simulink model "vsc_3w_l_filter"  (Simulink 8.9)
settings: Solver=ode23t  StartTime=0.0  StopTime=1  FixedStep=100.0e-6  RelTol=1e-6
values from neighbouring files (symbols this model uses):
  C_dc = 1e6    (= 1000000)    [ini_vsc_3w_l.m]
  F_b = 50.0    (= 50)    [ini_vsc_3w_l.m]
  K_i = R_s/tau_ref    (= 40)    [ini_vsc_3w_l.m]
  K_p = L_s/tau_ref    (= 0.5)    [ini_vsc_3w_l.m]
  L_s = 2.5e-3    (= 0.0025)    [ini_vsc_3w_l.m]
  R_s = 0.2    [ini_vsc_3w_l.m]
  V_dc = 730.0    (= 730)    [ini_vsc_3w_l.m]
  vsc_ctrl_ini = [0,0]    [ini_vsc_3w_l.m]
  vsc_ini = [0,0,V_dc]    [ini_vsc_3w_l.m]
libraries: powerlib x8, powerlib_meascontrol x3
settings Model: Creator=jmmauricio  LastModifiedBy=jmmauricio
settings SolverCC: AlgebraicLoopSolver=LineSearch
settings DataIOCC: LimitDataPoints=off  SaveFormat=Dataset  SignalLoggingSaveFormat=Dataset
settings DebuggingCC: UnderspecifiedInitializationDetection=Simplified  MergeDetectMultiDrivingBlocksExec=error  FcnCallInpInsideContextMsg=error  StateNameClashWarn=none  SFUnexpectedBacktrackingDiag=error  SFNoUnconditionalDefaultTransitionDiag=error
settings HardwareCC: ProdBitPerPointer=64  ProdBitPerSizeT=64  ProdBitPerPtrDiffT=64  ProdLargestAtomicFloat=Float  ProdIntDivRoundTo=Zero  ProdEndianess=LittleEndian  ProdWordSize=64  ProdHWDeviceType=Intel->x86-64 (Windows64)
settings ModelReferenceCC: PropagateSignalLabelsOutOfModel=on
settings GRTTargetCC: TargetLangStandard=C99 (ISO)  GeneratePreprocessorConditionals=Use local settings  CombineOutputUpdateFcns=on  GRTInterface=off
settings ConfigComp: CovMetricSettings=dwe  CovHtmlReporting=off  CovSaveCumulativeToWorkspaceVar=off  CovSaveSingleToWorkspaceVar=off  CovExternalEMLEnable=on

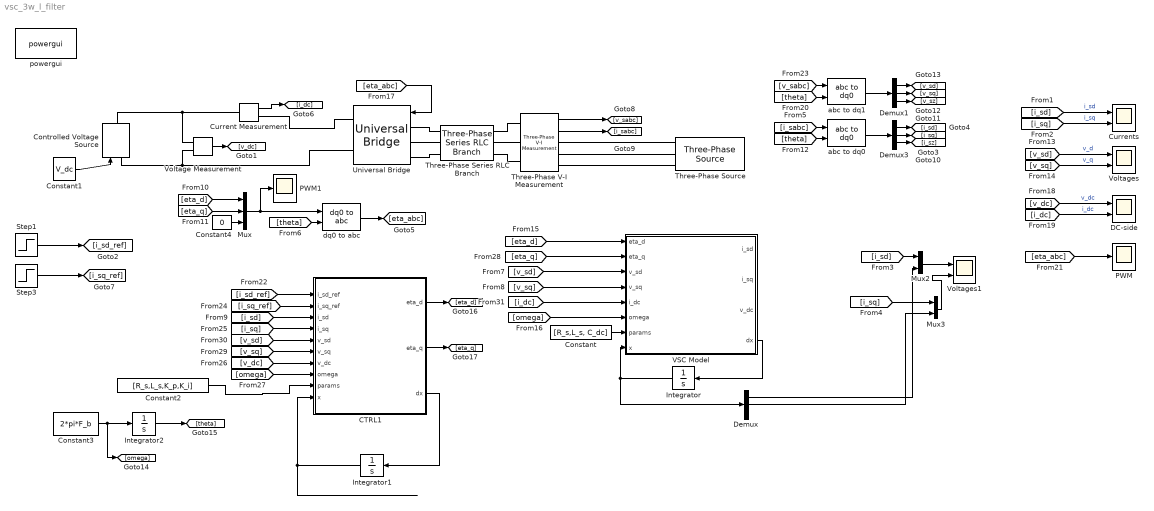
== system vsc_3w_l_filter ==
  CTRL1 : MATLAB Function  TreatAsAtomicUnit=on
  Constant : Constant  Value=[R_s,L_s, C_dc]
  Constant1 : Constant  Value=V_dc
  Constant2 : Constant  Value=[R_s,L_s,K_p,K_i]
  Constant3 : Constant  Value=2*pi*F_b
  Constant4 : Constant  Value=0
  Controlled Voltage Source : powerlib/Electrical Sources/Controlled Voltage Source  Initialize=on  Source_Type=AC  Amplitude=0  Phase=0  Frequency=0  Measurements=None
  Current Measurement : powerlib/Measurements/Current Measurement  PhasorSimulation=off  OutputType=Complex  PSBequivalent=0
  Currents : Scope  NumInputPorts=2
  DC-side : Scope  NumInputPorts=2
  Demux : Demux  Outputs=3
  Demux1 : Demux  Outputs=3
  Demux3 : Demux  Outputs=3
  Integrator : Integrator  InitialCondition=vsc_ini
  Integrator1 : Integrator  InitialCondition=vsc_ctrl_ini
  Integrator2 : Integrator
  Mux : Mux  Inputs=3
  Mux2 : Mux  Inputs=2
  Mux3 : Mux  Inputs=2
  PWM : Scope
  PWM1 : Scope
  Step1 : Step  Time=0.1  After=100  SampleTime=0
  Step3 : Step  Time=0.15  After=-100  SampleTime=0
  Three-Phase Series RLC Branch : powerlib/Elements/Three-Phase Series RLC Branch  LConnTagsString=A|B|C  RConnTagsString=A|B|C  BranchType=RL  Resistance=R_s  Inductance=L_s  Capacitance=1e-6  Measurements=None
  Three-Phase V-I Measurement : powerlib/Measurements/Three-Phase V-I Measurement  VoltageMeasurement=phase-to-ground  SetLabelV=off  LabelV=Vabc  Vpu=off  VpuLL=off  CurrentMeasurement=yes  SetLabelI=off  LabelI=Iabc  Ipu=off  Pbase=100e6  Vbase=500e3  OutputType=Complex  PhasorSimulation=off  PSBequivalent=0
  Three-Phase Source : powerlib/Electrical Sources/Three-Phase Source  InternalConnection=Yg  VoltagePhases=off  Voltage=400  PhaseAngle=0  Voltage_phases=[25e3 25e3 25e3]/sqrt(3)  PhaseAngles_phases=[0 -120 +120]  Frequency=50  NonIdealSource=off  SpecifyImpedance=off  Resistance=0.8929  Inductance=16.58e-3  ShortCircuitLevel=100e6  BaseVoltage=25e3  XRratio=7  BusType=swing  Pref=10e3  Qref=0  Prefabc=[10e3, 10e3, 10e3]  Qrefabc=[0, 0, 0]  Qmin=-inf  Qmax=inf
  Universal Bridge : powerlib/Power Electronics/Universal Bridge  Arms=3  SnubberResistance=1e5  SnubberCapacitance=inf  Device=Average-model based VSC  Ron=1e-3  Lon=0  ForwardVoltages="[  0  0  ]"  ForwardVoltage=0  GTOparameters=[ 10e-6 , 20e-6 ]  IGBTparameters=[ 1e-6 , 2e-6 ]  Measurements=None  Measurements_2=None  converterType=Rectifier
  VSC Model : MATLAB Function  TreatAsAtomicUnit=on
  Voltage Measurement : powerlib/Measurements/Voltage Measurement  PhasorSimulation=off  OutputType=Complex  PSBequivalent=0
  Voltages : Scope  NumInputPorts=2
  Voltages1 : Scope  NumInputPorts=2
  abc to dq0 : powerlib_meascontrol/Transformations/abc to dq0  Alignment=Aligned with phase A axis
  abc to dq1 : powerlib_meascontrol/Transformations/abc to dq0  Alignment=Aligned with phase A axis
  dq0 to abc : powerlib_meascontrol/Transformations/dq0 to abc  Alignment=Aligned with phase A axis
  powergui : powerlib/powergui  Priority=1  SimulationMode=Continuous  SampleTime=50e-6  frequency=60  Iterations=50  frequencyindice=0  Pbase=100e6  ErrMax=1e-4  UnitsV=kV  UnitsW=MW  buscounter=0  FunctionMessages=off  echomessages=off  EnableUseOfTLC=off  CurrentSourceSwitches=off  DisableSnubberDevices=off  DisableRonSwitches=off  DisableVfSwitches=off  DisplayEquations=off  SolverType=Tustin/Backward Euler (TBE)  Interpol=off  ExternalGateDelay=off  methode=off  Ts=100  x0status=blocks  SPID=on  SwTol=0  HookPort=off  RestoreLinks=warning  ResistiveCurrentMeasurement=off  Frange=[0:2:500]  Ylog=off  Xlog=on  ShowGrid=off  save=off  variable=ZData  structure=0  ZoomFFT=off  StartTime=0.0  cycles=1  DisplayStyle=1  fundamental=60  FreqAxis=off  MaxFrequency=1000  frequencyindicesteady=1  RmsSteady=1  display=off
  wires:
  Integrator/1 -> VSC Model/8(x), Demux/1
  Constant/1 -> VSC Model/7(params)
  VSC Model/4(dx) -> Integrator/1
  [omega] -> VSC Model/6(omega)
  Mux/1 -> PWM1/1, dq0 to abc/1
  [i_sd] -> Currents/1  "i_sd"
  [theta] -> dq0 to abc/2
  [v_sd] -> VSC Model/3(v_sd)
  [v_sq] -> VSC Model/4(v_sq)
  [eta_d] -> Mux/1
  [eta_q] -> Mux/2
  abc to dq0/1 -> Demux3/1
  Demux3/1 -> [i_sd]
  Demux3/2 -> [i_sq]
  [v_sd] -> Voltages/1  "v_d"
  [v_sq] -> Voltages/2  "v_q"
  [eta_abc] -> Universal Bridge/1
  Constant4/1 -> Mux/3
  Voltage Measurement/1 -> [v_dc]
  [v_dc] -> DC-side/1  "v_dc"
  Current Measurement/1 -> [i_dc]
  [i_dc] -> DC-side/2  "i_dc"
  [i_sq] -> Currents/2  "i_sq"
  [eta_abc] -> PWM/1
  Constant1/1 -> Controlled Voltage Source/1
  Mux2/1 -> Voltages1/1
  Mux3/1 -> Voltages1/2
  Demux/1 -> Mux2/2
  [i_sd] -> Mux2/1
  Demux/2 -> Mux3/2
  Step1/1 -> [i_sd_ref]
  Step3/1 -> [i_sq_ref]
  [i_sq_ref] -> CTRL1/2(i_sq_ref)
  [i_sd_ref] -> CTRL1/1(i_sd_ref)
  [i_sd] -> CTRL1/3(i_sd)
  CTRL1/3(dx) -> Integrator1/1
  Constant2/1 -> CTRL1/9(params)
  Integrator1/1 -> CTRL1/10(x)
  [i_sq] -> CTRL1/4(i_sq)
  [v_dc] -> CTRL1/7(v_dc)
  [omega] -> CTRL1/8(omega)
  Three-Phase V-I Measurement/1 -> [v_sabc]
  Three-Phase V-I Measurement/2 -> [i_sabc]
  [i_sabc] -> abc to dq0/1
  [theta] -> abc to dq0/2
  Demux3/3 -> [i_sz]
  Demux1/3 -> [v_sz]
  [theta] -> abc to dq1/2
  [v_sabc] -> abc to dq1/1
  Demux1/2 -> [v_sq]
  Demux1/1 -> [v_sd]
  abc to dq1/1 -> Demux1/1
  Constant3/1 -> [omega], Integrator2/1
  Integrator2/1 -> [theta]
  CTRL1/1(eta_d) -> [eta_d]
  CTRL1/2(eta_q) -> [eta_q]
  [eta_q] -> VSC Model/2(eta_q)
  [eta_d] -> VSC Model/1(eta_d)
  [v_sq] -> CTRL1/6(v_sq)
  [v_sd] -> CTRL1/5(v_sd)
  [i_dc] -> VSC Model/5(i_dc)
  dq0 to abc/1 -> [eta_abc]
  [i_sq] -> Mux3/1
  connections:
  Three-Phase Series RLC Branch/LConn1 -- Universal Bridge/LConn1
  Three-Phase Series RLC Branch/LConn3 -- Universal Bridge/LConn3
  Three-Phase Series RLC Branch/LConn2 -- Universal Bridge/LConn2
  Voltage Measurement/LConn2 -- Controlled Voltage Source/LConn1 -- Universal Bridge/RConn2
  Current Measurement/RConn1 -- Universal Bridge/RConn1
  Current Measurement/LConn1 -- Voltage Measurement/LConn1 -- Controlled Voltage Source/RConn1
  Three-Phase V-I Measurement/LConn2 -- Three-Phase Series RLC Branch/RConn2
  Three-Phase Series RLC Branch/RConn1 -- Three-Phase V-I Measurement/LConn1
  Three-Phase Series RLC Branch/RConn3 -- Three-Phase V-I Measurement/LConn3
  Three-Phase Source/RConn3 -- Three-Phase V-I Measurement/RConn3
  Three-Phase Source/RConn2 -- Three-Phase V-I Measurement/RConn2
  Three-Phase Source/RConn1 -- Three-Phase V-I Measurement/RConn1

== matlab function CTRL1 ==
  data: eta_d output double; eta_q output double; i_sd_ref input double; i_sq_ref input double; i_sd input double; i_sq input double; v_sd input double; v_sq input double; v_dc input double; omega input double; params input double; dx output double; x input double
function [eta_d,eta_q,dx] = ctrl_vsc(i_sd_ref,i_sq_ref,i_sd,i_sq,v_sd,v_sq,v_dc,omega,params,x)

% parameters
R_s = params(1);
L_s = params(2);
K_p = params(3);
K_i = params(4);

% from the integrator to the states
xi_isd  = x(1);
xi_isq  = x(2);


% auxiliar
e_isd =  i_sd_ref - i_sd;
e_isq =  i_sq_ref - i_sq;


% derivatives
dxi_isd  = e_isd;
dxi_isq  = e_isq;


% auxiliar
u_d = K_p*e_isd + K_i*xi_isd;
u_q = K_p*e_isq + K_i*xi_isq;

% outputs
eta_d  = 2 / v_dc * ( u_d  - L_s * omega * i_sq  + v_sd);
eta_q  = 2 / v_dc * ( u_q  + L_s * omega * i_sd  + v_sq);


% from derivatives to the integrator
dx = [dxi_isd,dxi_isq];

== matlab function VSC Model ==
  data: eta_d input double; eta_q input double; i_sd output double; i_sq output double; v_dc output double; v_sd input double; v_sq input double; i_dc input double; omega input double; params input double; dx output double; x input double
function [i_sd,i_sq,v_dc,dx] = vsc_l_dq(eta_d,eta_q,v_sd,v_sq,i_dc,omega,params,x)

% parameters
R_s  = params(1);
L_s  = params(2);
C_dc = params(3);

% from the integrator to the states
i_sd  = x(1);
i_sq  = x(2);
v_dc =  x(3);

% derivatives
di_sd  = 1/L_s*(0.5*eta_d*v_dc + L_s*omega*i_sq - R_s*i_sd - v_sd);
di_sq  = 1/L_s*(0.5*eta_q*v_dc - L_s*omega*i_sd - R_s*i_sq - v_sq);
dv_dc = 1/C_dc * ( 0.5 * (eta_d *i_sd  + eta_q * i_sq  - i_dc ));

% from derivatives to the integrator
dx = [di_sd,di_sq,dv_dc];
